simulink model "idcs_gimbal_plant"  (R2026a)
settings: Solver=ode4  StopTime=5  FixedStep=0.01
settings Model: Creator=2681a  LastModifiedBy=2681a

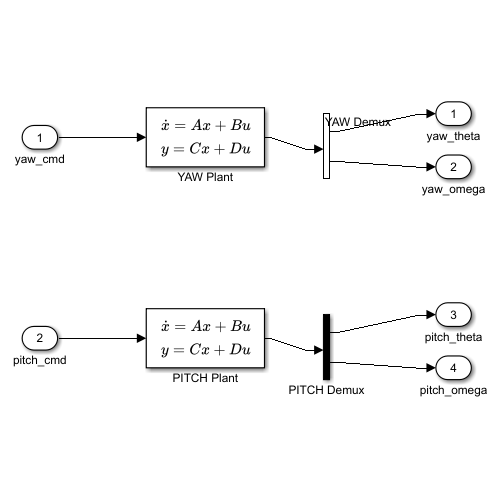
[thumbnail: Simulink's stored preview of the top-level diagram]
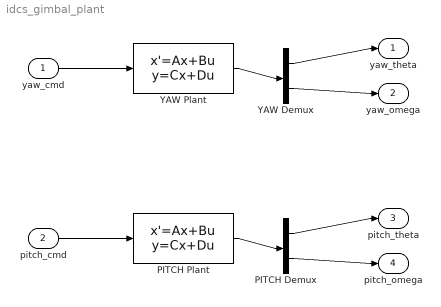
== system idcs_gimbal_plant ==
  yaw_cmd : Inport
  pitch_cmd : Inport  Port=2
  PITCH Demux : Demux  Outputs=2
  PITCH Plant : StateSpace  A=[0 1; 0 -12.773593392785243]  B=[0; 11.732636074122547]  C=[1 0; 0 1]  D=[0; 0]  InitialCondition=0
  YAW Demux : Demux  Outputs=2
  YAW Plant : StateSpace  A=[0 1; 0 -13.278338106322355]  B=[0; 13.24929867571994]  C=[1 0; 0 1]  D=[0; 0]  InitialCondition=0
  yaw_theta : Outport
  yaw_omega : Outport  Port=2
  pitch_theta : Outport  Port=3
  pitch_omega : Outport  Port=4
  wires:
  yaw_cmd/1 -> YAW Plant/1
  YAW Plant/1 -> YAW Demux/1
  YAW Demux/1 -> yaw_theta/1
  YAW Demux/2 -> yaw_omega/1
  pitch_cmd/1 -> PITCH Plant/1
  PITCH Plant/1 -> PITCH Demux/1
  PITCH Demux/1 -> pitch_theta/1
  PITCH Demux/2 -> pitch_omega/1
